simulink model "fig7_73ol"  (Simulink 6.1)
settings: Solver=ode23  StartTime=0.0  StopTime=300.0  RelTol=1e-6
settings Model: LastModifiedBy=abbas  ExtModeTrigMode=oneshot  ExtModeArmWhenConnect=off
settings DataIOCC: LimitDataPoints=off
settings OptimizationCC: BlockReduction=off  BooleanDataType=off
settings HardwareCC: TargetUnknown=on
settings STFCustomTargetCC: TargetFcnLib=ansi_tfl_tmw.mat  GenFloatMathFcnCalls=ANSI_C  ModelReferenceCompliant=off  SystemTargetFile=grt.tlc

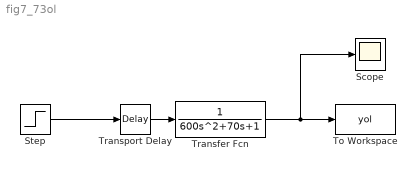
== system fig7_73ol ==
  Scope : Scope
  Step : Step  SampleTime=0
  To Workspace : ToWorkspace  VariableName=yol  SampleTime=-1  SaveFormat=Array
  Transfer Fcn : TransferFcn  Denominator=[600 70 1]
  Transport Delay : TransportDelay  DelayTime=5
  wires:
  Transport Delay/1 -> Transfer Fcn/1
  Transfer Fcn/1 -> To Workspace/1, Scope/1
  Step/1 -> Transport Delay/1
